simulink model "model_surge"  (R2014a)
settings: Solver=ode45  StartTime=0.0  StopTime=8000  RelTol=1e-3
settings Model: Creator=Mat  LastModifiedBy=Hwk
settings DebuggingCC: UnderspecifiedInitializationDetection=Classic  StateNameClashWarn=warning

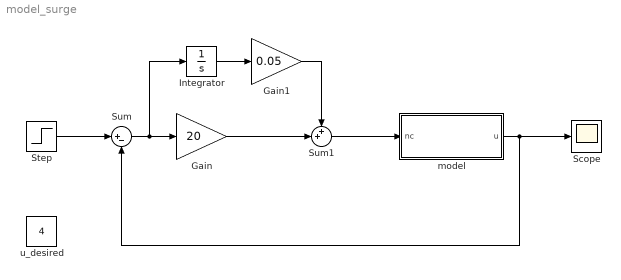
== system model_surge ==
  Gain : Gain  Gain=20
  Gain1 : Gain  Gain=0.05
  Integrator : Integrator
  Scope : Scope
      settings: TimeRange=8000  YMin=0  YMax=7
  Step : Step  Time=0  After=7.3  SampleTime=0
  Sum : Sum  Inputs=|+-
  Sum1 : Sum  Inputs=++|
  model : Subsystem
  u_desired : Constant  Value=4
  wires:
  model/1(u) -> Sum/2, Scope/1
  Sum/1 -> Integrator/1, Gain/1
  Gain/1 -> Sum1/2
  Gain1/1 -> Sum1/1
  Sum1/1 -> model/1(nc)
  Step/1 -> Sum/1
  Integrator/1 -> Gain1/1

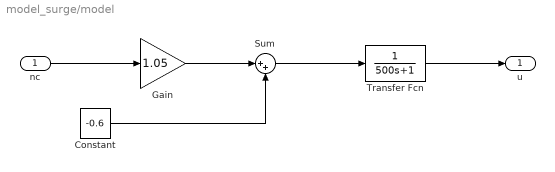
== system model_surge/model ==
  nc : Inport
  Constant : Constant  Value=-0.6
  Gain : Gain  Gain=1.05
  Sum : Sum  Inputs=|++
  Transfer Fcn : TransferFcn  Denominator=[500 1]
  u : Outport
  wires:
  nc/1 -> Gain/1
  Constant/1 -> Sum/2
  Gain/1 -> Sum/1
  Sum/1 -> Transfer Fcn/1
  Transfer Fcn/1 -> u/1
